simulink model "first_simulink"  (R2020a)
settings: Solver=VariableStepAuto  StartTime=0.0  StopTime=10.0  RelTol=1e-3
settings Model: Creator=Francesco  LastModifiedBy=Francesco

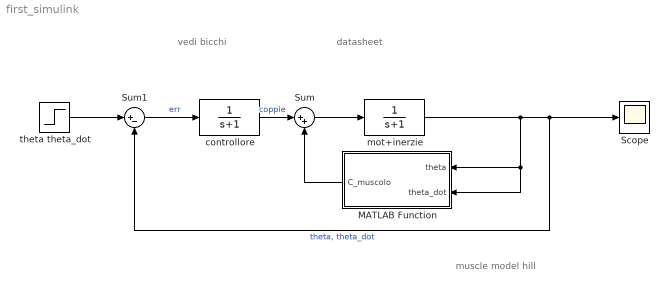
== system first_simulink ==
  note: muscle model hill
  note: datasheet
  note: vedi bicchi
  MATLAB Function : MATLAB Function  TreatAsAtomicUnit=on
  Scope : Scope
  Sum : Sum  Inputs=|++
  Sum1 : Sum  Inputs=|+-
  controllore : TransferFcn  Denominator=[1 1]
  mot+inerzie : TransferFcn  Denominator=[1 1]
  theta theta_dot : Step  SampleTime=0
  wires:
  mot+inerzie/1 -> MATLAB Function/1(theta), MATLAB Function/2(theta_dot), Sum1/2, Scope/1  "theta, theta_dot"
  MATLAB Function/1(C_muscolo) -> Sum/2
  Sum/1 -> mot+inerzie/1
  Sum1/1 -> controllore/1  "err"
  theta theta_dot/1 -> Sum1/1
  controllore/1 -> Sum/1  "coppie"

== matlab function first_simulink/MATLAB Function ==
  data: theta input; C_muscolo output; theta_dot input
function C_muscolo = fcn(theta, theta_dot)

y = u;
